simulink model "cross_track"  (Simulink 7.1)
settings: Solver=ode4  StartTime=0.0  StopTime=1500  FixedStep=0.1  RelTol=1e-3
libraries: fordypningsprosjekt x3, simulink x1
settings Model: Creator=anderga  LastModifiedBy=anders

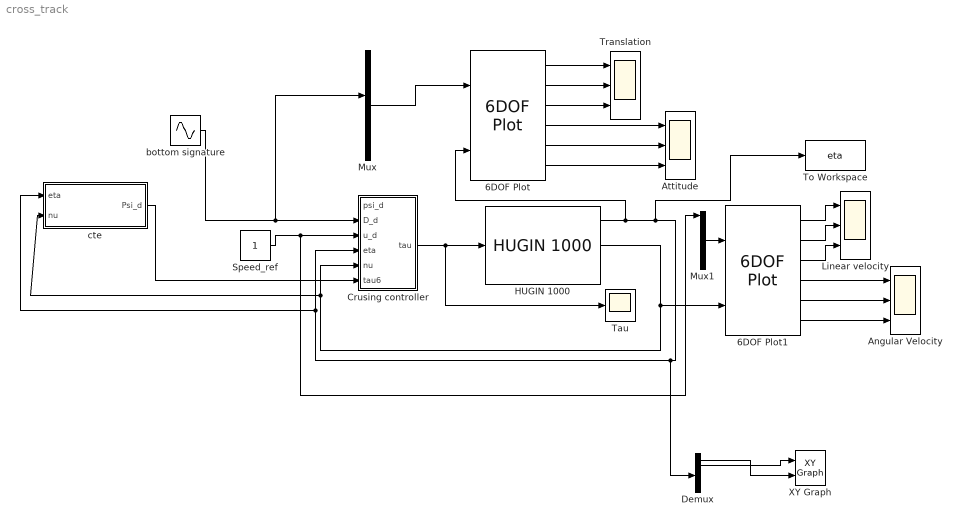
== system cross_track ==
  6DOF Plot : fordypningsprosjekt/6DOF Plot  SystemSampleTime=-1
  6DOF Plot1 : fordypningsprosjekt/6DOF Plot  SystemSampleTime=-1
  Angular Velocity : Scope  NumInputPorts=3
      settings: YMin=-3.5~-4.5~-40  YMax=0.5~0.5~5  SaveName=ScopeData3
  Attitude : Scope  NumInputPorts=3
      settings: YMin=-7~-25~0  YMax=1~5~90  SaveName=Attitude_ref
  Crusing controller : Subsystem  AncestorBlock=fordypningsprosjekt/Crusing controller  mask{Kp_u=10, Ki_u=3, Kp_c=400, Kd_c=200, Kp_d=5, Kp2_d=3, Kd_d=4}
      mask prompts: Kp_u "Kp Speed controller"; Ki_u "Ki Speed Controller"; Kp_c "Kp Course Controller"; Kd_c "Kd Course Controller"; Kp_d "Kp1 Depth Controller"; Kp2_d "Kp2 Depth controller"; Kd_d "Kd Depth Controller"
  Demux : Demux  Outputs=6
  HUGIN 1000 : fordypningsprosjekt/HUGIN 1000  SystemSampleTime=-1  eta_0=[0 10 0 0 0 pi/6]  nu_0=[0 0 0 0 0 0]  c_on_off=off  beta_c=45  V_c=0.3
  Linear velocity : Scope  NumInputPorts=3
      settings: YMin=0~-0.6~-0.025  YMax=1.75~0.2~0.3  SaveName=ScopeData2
  Mux : Mux  Inputs=6
  Mux1 : Mux  Inputs=6
  Speed_ref : Constant  OutDataType=sfix(16)  OutScaling=2^0
  Tau : Scope
      settings: YMin=-600  YMax=600  SaveName=ScopeData4
  To Workspace : ToWorkspace  VariableName=eta  SampleTime=-1  SaveFormat=Structure With Time
  Translation : Scope  NumInputPorts=3
      settings: YMin=-800~-40~0  YMax=100~60~60  SaveName=Translation_ref
  XY Graph : simulink/Sinks/XY Graph  SystemSampleTime=-1  xmin=-1000  xmax=1000  ymin=-1000  ymax=1000  st=-1
  bottom signature : Sin  Amplitude=6  Bias=50  Frequency=0.01  SampleTime=0
  cte : Subsystem
  wires:
  Crusing controller/1(tau) -> HUGIN 1000/1, Tau/1
  HUGIN 1000/1 -> 6DOF Plot/2, Crusing controller/4(eta), cte/1(eta), Demux/1, To Workspace/1
  HUGIN 1000/2 -> Crusing controller/5(nu), cte/2(nu), 6DOF Plot1/2
  bottom signature/1 -> Crusing controller/2(D_d), Mux/3
  Speed_ref/1 -> Crusing controller/3(u_d), Mux1/1
  cte/1(Psi_d) -> Crusing controller/6(tau6)
  Mux/1 -> 6DOF Plot/1
  6DOF Plot/1 -> Translation/1
  6DOF Plot/2 -> Translation/2
  6DOF Plot/3 -> Translation/3
  6DOF Plot/4 -> Attitude/1
  6DOF Plot/5 -> Attitude/2
  6DOF Plot/6 -> Attitude/3
  Mux1/1 -> 6DOF Plot1/1
  6DOF Plot1/1 -> Linear velocity/1
  6DOF Plot1/2 -> Linear velocity/2
  6DOF Plot1/3 -> Linear velocity/3
  6DOF Plot1/4 -> Angular Velocity/1
  6DOF Plot1/5 -> Angular Velocity/2
  6DOF Plot1/6 -> Angular Velocity/3
  Demux/1 -> XY Graph/2
  Demux/2 -> XY Graph/1

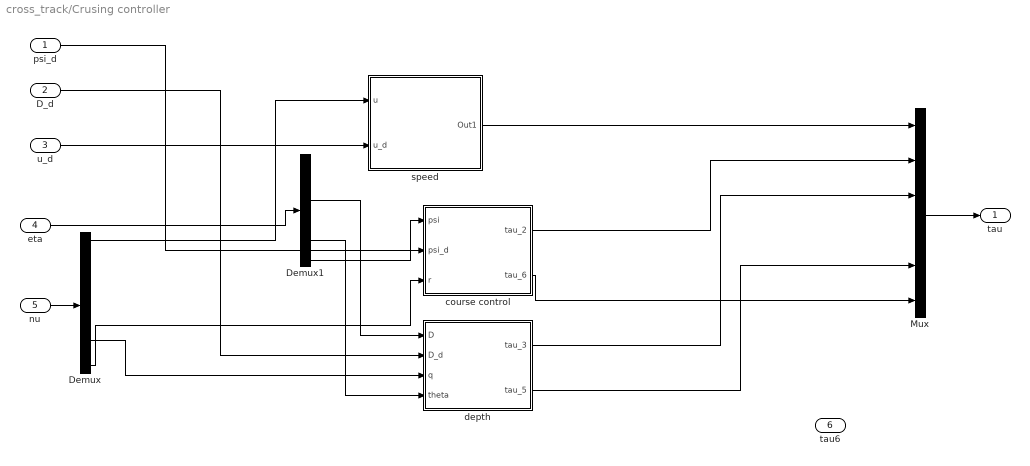
== system cross_track/Crusing controller ==
  psi_d : Inport  OutDataType=sfix(16)  OutScaling=2^0
  D_d : Inport  Port=2  OutDataType=sfix(16)  OutScaling=2^0
  u_d : Inport  Port=3  OutDataType=sfix(16)  OutScaling=2^0
  eta : Inport  Port=4  OutDataType=sfix(16)  OutScaling=2^0
  nu : Inport  Port=5  OutDataType=sfix(16)  OutScaling=2^0
  tau6 : Inport  Port=6  OutDataType=sfix(16)  OutScaling=2^0
  Demux : Demux  Outputs=6
  Demux1 : Demux  Outputs=6
  Mux : Mux  Inputs=6
  course control : Subsystem
  depth : Subsystem
  speed : Subsystem
  tau : Outport  OutDataType=sfix(16)  OutScaling=2^0
  wires:
  nu/1 -> Demux/1
  Demux/1 -> speed/1(u)
  u_d/1 -> speed/2(u_d)
  eta/1 -> Demux1/1
  Demux1/6 -> course control/1(psi)
  psi_d/1 -> course control/2(psi_d)
  Demux/6 -> course control/3(r)
  speed/1(Out1) -> Mux/1
  Mux/1 -> tau/1
  D_d/1 -> depth/2(D_d)
  Demux1/3 -> depth/1(D)
  Demux/5 -> depth/3(q)
  Demux1/5 -> depth/4(theta)
  depth/1(tau_3) -> Mux/3
  depth/2(tau_5) -> Mux/5
  course control/1(tau_2) -> Mux/2
  course control/2(tau_6) -> Mux/6

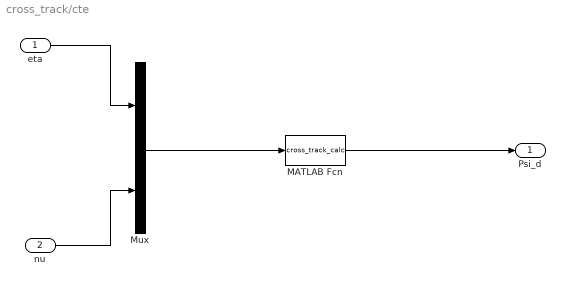
== system cross_track/cte ==
  eta : Inport  OutDataType=sfix(16)  OutScaling=2^0
  nu : Inport  Port=2  OutDataType=sfix(16)  OutScaling=2^0
  MATLAB Fcn : MATLABFcn  MATLABFcn=cross_track_calc  OutputDimensions=1
  Mux : Mux  Inputs=2
  Psi_d : Outport  OutDataType=sfix(16)  OutScaling=2^0
  wires:
  eta/1 -> Mux/1
  nu/1 -> Mux/2
  Mux/1 -> MATLAB Fcn/1
  MATLAB Fcn/1 -> Psi_d/1

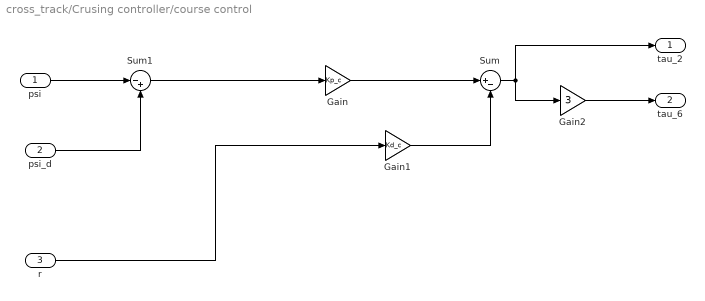
== system cross_track/Crusing controller/course control ==
  psi : Inport  OutDataType=sfix(16)  OutScaling=2^0
  psi_d : Inport  Port=2  OutDataType=sfix(16)  OutScaling=2^0
  r : Inport  Port=3  OutDataType=sfix(16)  OutScaling=2^0
  Gain : Gain  Gain=Kp_c  ParameterDataType=sfix(16)  ParameterScaling=2^0  OutDataType=sfix(16)  OutScaling=2^0
  Gain1 : Gain  Gain=Kd_c  ParameterDataType=sfix(16)  ParameterScaling=2^0  OutDataType=sfix(16)  OutScaling=2^0
  Gain2 : Gain  Gain=3  ParameterDataType=sfix(16)  ParameterScaling=2^0  OutDataType=sfix(16)  OutScaling=2^0
  Sum : Sum  Inputs=|+-  OutDataType=sfix(16)  OutScaling=2^0
  Sum1 : Sum  Inputs=|-+  OutDataType=sfix(16)  OutScaling=2^0
  tau_2 : Outport  OutDataType=sfix(16)  OutScaling=2^0
  tau_6 : Outport  Port=2  OutDataType=sfix(16)  OutScaling=2^0
  wires:
  Sum1/1 -> Gain/1
  Gain1/1 -> Sum/2
  psi/1 -> Sum1/1
  psi_d/1 -> Sum1/2
  Gain/1 -> Sum/1
  r/1 -> Gain1/1
  Sum/1 -> Gain2/1, tau_2/1
  Gain2/1 -> tau_6/1

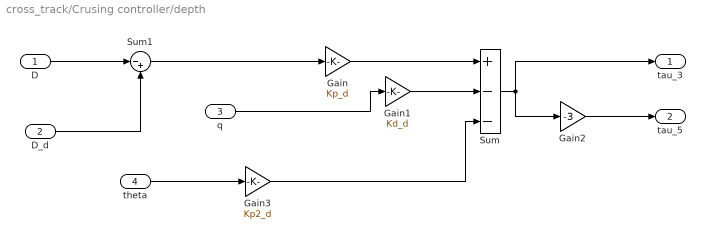
== system cross_track/Crusing controller/depth ==
  D : Inport  OutDataType=sfix(16)  OutScaling=2^0
  D_d : Inport  Port=2  OutDataType=sfix(16)  OutScaling=2^0
  q : Inport  Port=3  OutDataType=sfix(16)  OutScaling=2^0
  theta : Inport  Port=4  OutDataType=sfix(16)  OutScaling=2^0
  Gain : Gain  Gain=Kp_d  ParameterDataType=sfix(16)  ParameterScaling=2^0  OutDataType=sfix(16)  OutScaling=2^0
  Gain1 : Gain  Gain=Kd_d  ParameterDataType=sfix(16)  ParameterScaling=2^0  OutDataType=sfix(16)  OutScaling=2^0
  Gain2 : Gain  Gain=-3  ParameterDataType=sfix(16)  ParameterScaling=2^0  OutDataType=sfix(16)  OutScaling=2^0
  Gain3 : Gain  Gain=Kp2_d  ParameterDataType=sfix(16)  ParameterScaling=2^0  OutDataType=sfix(16)  OutScaling=2^0
  Sum : Sum  Inputs=+--  OutDataType=sfix(16)  OutScaling=2^0
  Sum1 : Sum  Inputs=|-+  OutDataType=sfix(16)  OutScaling=2^0
  tau_3 : Outport  OutDataType=sfix(16)  OutScaling=2^0
  tau_5 : Outport  Port=2  OutDataType=sfix(16)  OutScaling=2^0
  wires:
  Gain2/1 -> tau_5/1
  Sum/1 -> tau_3/1, Gain2/1
  q/1 -> Gain1/1
  Gain/1 -> Sum/1
  D_d/1 -> Sum1/2
  D/1 -> Sum1/1
  Gain1/1 -> Sum/2
  Sum1/1 -> Gain/1
  theta/1 -> Gain3/1
  Gain3/1 -> Sum/3

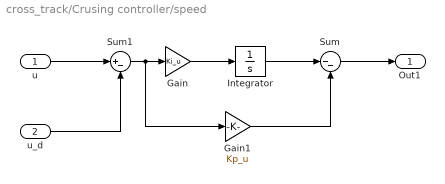
== system cross_track/Crusing controller/speed ==
  u : Inport  OutDataType=sfix(16)  OutScaling=2^0
  u_d : Inport  Port=2  OutDataType=sfix(16)  OutScaling=2^0
  Gain : Gain  Gain=Ki_u  ParameterDataType=sfix(16)  ParameterScaling=2^0  OutDataType=sfix(16)  OutScaling=2^0
  Gain1 : Gain  Gain=Kp_u  ParameterDataType=sfix(16)  ParameterScaling=2^0  OutDataType=sfix(16)  OutScaling=2^0
  Integrator : Integrator
  Sum : Sum  Inputs=|--  OutDataType=sfix(16)  OutScaling=2^0
  Sum1 : Sum  Inputs=|+-  OutDataType=sfix(16)  OutScaling=2^0
  Out1 : Outport  OutDataType=sfix(16)  OutScaling=2^0
  wires:
  Sum/1 -> Out1/1
  u/1 -> Sum1/1
  u_d/1 -> Sum1/2
  Sum1/1 -> Gain/1, Gain1/1
  Integrator/1 -> Sum/1
  Gain/1 -> Integrator/1
  Gain1/1 -> Sum/2
